simulink model "motor_sensor_PID"  (R2024b)
settings: Solver=FixedStepAuto  StartTime=0.0  StopTime=5  RelTol=1e-3  EnableMultiTasking=on
libraries: arduinolib x4, slpidlib x1, arduinosensorlib x1
settings Model: ExtModeTrigDuration=2  Creator=The MathWorks, Inc.  LastModifiedBy=davil
settings SolverCC: AlgebraicLoopSolver=TrustRegion  AutoInsertRateTranBlk=on
settings DataIOCC: ReturnWorkspaceOutputs=off
settings OptimizationCC: PassReuseOutputArgsThreshold=0  MaxStackSize=64
settings DebuggingCC: ParameterTunabilityLossMsg=error  UnconnectedInputMsg=warning  UnconnectedOutputMsg=warning  UnconnectedLineMsg=warning  ArithmeticOperatorsInVariantConditions=warning
settings HardwareCC: ProdBitPerInt=16  ProdBitPerPointer=16  ProdBitPerSizeT=16  ProdBitPerPtrDiffT=16  ProdLargestAtomicFloat=None  ProdWordSize=8  ProdHWDeviceType=Atmel->AVR  UseEmbeddedCoderFeatures=off  UseSimulinkCoderFeatures=off
settings ModelReferenceCC: EnableRefExpFcnMdlSchedulingChecks=on
settings SFSimCC: SimUseLocalCustomCode=off  MATLABDynamicMemAlloc=off  CustomCodeUndefinedFunction=UseInterfaceOnly
settings RTWCC: Description=Embedded Coder  SystemTargetFile=ert.tlc  HardwareBoard=Arduino Uno  TemplateMakefile=ert_default_tmf  GenerateReport=on  RTWUseLocalCustomCode=off  Toolchain=Arduino AVR  BuildConfiguration=Faster Runs  LaunchReport=on  GPUComputeCapability=3.5
settings CodeAppCC: ForceParamTrailComments=on  OperatorAnnotations=on
settings ERTTargetCC: ERTCustomFileBanners=off  SupportContinuousTime=on  SupportNonInlinedSFcns=on  RemoveResetFunc=off  SupportVariableSizeSignals=on  ModelStepFunctionPrototypeControlCompliant=off  ExtModeTransport=3  ExtModeStaticAlloc=on  ExtModeAutomaticAllocSize=off  ExtModeStaticAllocSize=250  ExtModeMexFile=ext_xcp  ExtModeIntrfLevel=Level2 - Open  InlinedParameterPlacement=Hierarchical  DynamicArrayContainerType=coder::array

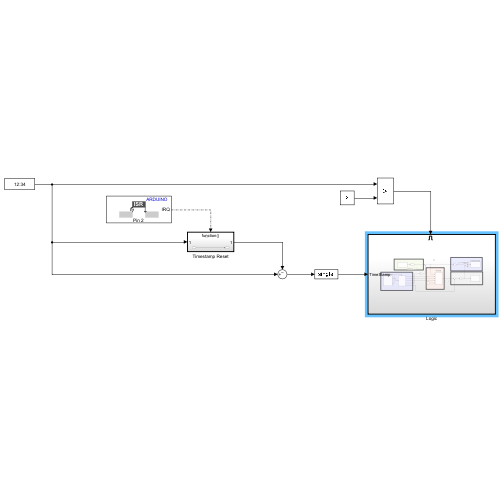
[thumbnail: Simulink's stored preview of the top-level diagram]
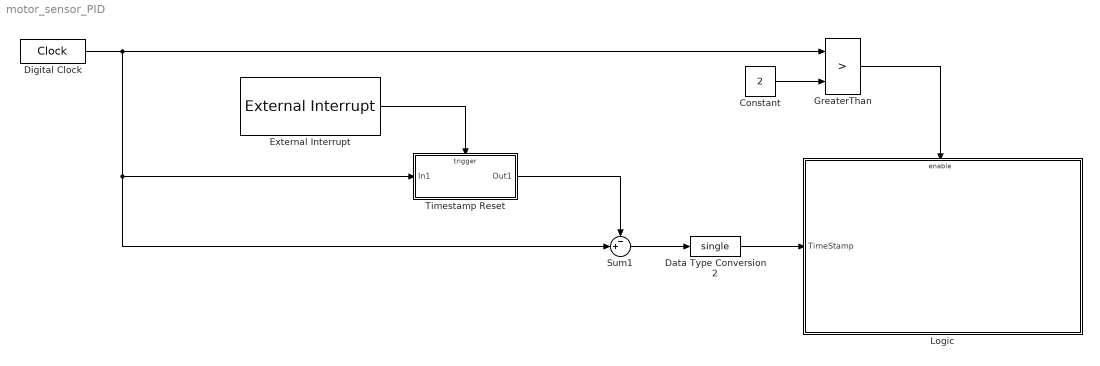
== system motor_sensor_PID ==
  Constant : Constant  Value=2
  Data Type Conversion2 : DataTypeConversion  OutDataTypeStr=single  RndMeth=Round  SaturateOnIntegerOverflow=off
  Digital Clock : DigitalClock  SampleTime=0.1
  External Interrupt : arduinolib/External Interrupt  Pin=2  PullUp=off  Mode=RISING  InterruptSimulationInput=off
  GreaterThan : RelationalOperator  Operator=>  OutDataTypeStr=boolean  RndMeth=Simplest  InputSameDT=off
  Logic : Subsystem
  Sum1 : Sum  Inputs=-+|
  Timestamp Reset : Subsystem  TreatAsAtomicUnit=on
  wires:
  GreaterThan/1 -> Logic/Enable
  Constant/1 -> GreaterThan/2
  Digital Clock/1 -> GreaterThan/1, Timestamp Reset/1(In1), Sum1/2
  Sum1/1 -> Data Type Conversion2/1
  Timestamp Reset/1(Out1) -> Sum1/1
  External Interrupt/1 -> Timestamp Reset/Trigger
  Data Type Conversion2/1 -> Logic/1(TimeStamp)

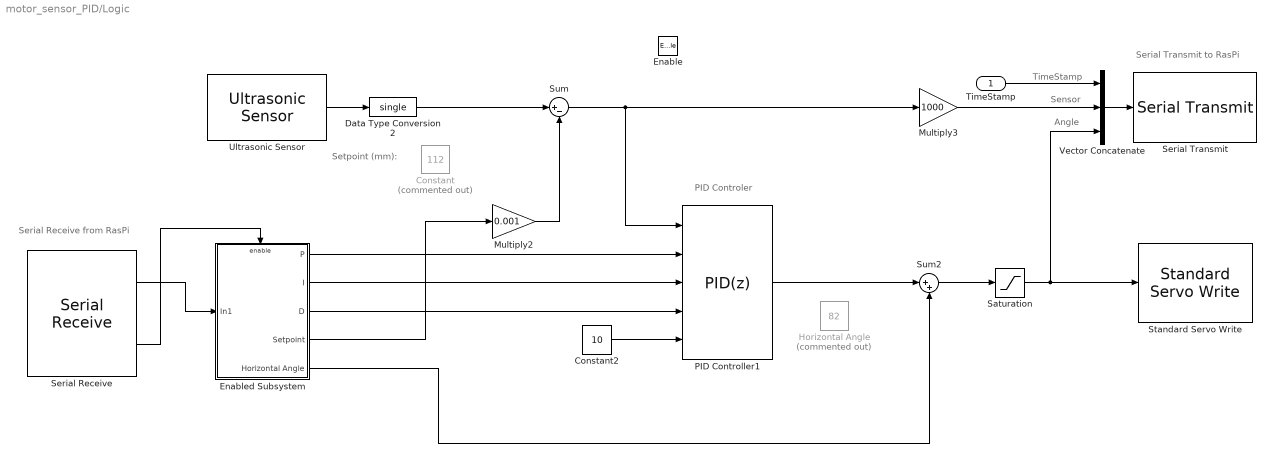
== system motor_sensor_PID/Logic ==
  note: Setpoint (mm):
  note: Serial Receive from RasPi
  note: PID Controler
  note: Serial Transmit to RasPi
  note: TimeStamp
  note: Sensor
  note: Angle
  TimeStamp : Inport
  Enable : EnablePort
  Constant : Constant  Commented=on  Value=112  OutDataTypeStr=single
  Constant2 : Constant  Value=10  OutDataTypeStr=single
  Data Type Conversion2 : DataTypeConversion  OutDataTypeStr=single  RndMeth=Round  SaturateOnIntegerOverflow=off
  Enabled Subsystem : Subsystem  TreatAsAtomicUnit=on
  Horizontal Angle : Constant  Commented=on  Value=82  OutDataTypeStr=single
  Multiply2 : Gain  Gain=0.001
  Multiply3 : Gain  Gain=1000
  PID Controller1 : slpidlib/PID Controller  Controller=PID  Form=Parallel  TimeDomain=Discrete-time  UseExternalTs=off  SampleTime=-1  IntegratorMethod=Forward Euler  FilterMethod=Forward Euler  ControllerParametersSource=external  P=1  I=1  UseKiTs=off  D=0  UseExternalDerivativeSource=off  N=100  UseFilter=on  TunerSelectOption=Transfer Function Based (PID Tuner App)  InitialConditionSource=internal  InitialConditionForIntegrator=0  InitialConditionForFilter=0  DifferentiatorICPrevScaledInput=0  ExternalReset=none  TrackingMode=off  Kt=1  LimitOutput=off  SatLimitsSource=internal  UpperSaturationLimit=180  LowerSaturationLimit=0  LinearizeAsGain=on  AntiWindupMode=none  Kb=1  LimitIntegrator=off  UpperIntegratorSaturationLimit=inf  LowerIntegratorSaturationLimit=-inf  POutMin=[]  POutMax=[]  IOutMin=[]  IOutMax=[]  DOutMin=[]  DOutMax=[]  NOutMin=[]  NOutMax=[]  SumOutMin=[]  SumOutMax=[]  SaturationOutMin=[]  SaturationOutMax=[]  PParamMin=[]  PParamMax=[]  IParamMin=[]  IParamMax=[]  DParamMin=[]  DParamMax=[]  NParamMin=[]  NParamMax=[]  KbParamMin=[]  KbParamMax=[]  KtParamMin=[]  KtParamMax=[]  KbOutMin=[]  KbOutMax=[]  KtOutMin=[]  KtOutMax=[]  IntegratorOutMin=[]  IntegratorOutMax=[]  FilterOutMin=[]  FilterOutMax=[]  SumI1OutMin=[]  SumI1OutMax=[]  SumI2OutMin=[]  SumI2OutMax=[]  SumI3OutMin=[]  SumI3OutMax=[]  SumI4OutMin=[]  SumI4OutMax=[]  SumDOutMin=[]  SumDOutMax=[]  DifferentiatorOutMin=[]  DifferentiatorOutMax=[]  FilterDiffOutCoefMin=[]  FilterDiffOutCoefMax=[]  ReciprocalOutMin=[]  ReciprocalOutMax=[]  SumDenOutMin=[]  SumDenOutMax=[]  SumNumOutMin=[]  SumNumOutMax=[]  DivideOutMin=[]  DivideOutMax=[]  UdiffTsProdOutMin=[]  UdiffTsProdOutMax=[]  NTsProdOutMin=[]  NTsProdOutMax=[]  UintegralTsProdOutMin=[]  UintegralTsProdOutMax=[]  UngainTsProdOutMin=[]  UngainTsProdOutMax=[]  ClampingZeroOutDataTypeStr=Inherit: Inherit via back propagation  ClampingZeroOutMin=[]  ClampingZeroOutMax=[]  FilterDenConstantOutDataTypeStr=Inherit: Inherit via back propagation  FilterDenConstantOutMin=[]  FilterDenConstantOutMax=[]  PCopyOutDataTypeStr=Inherit: Inherit via back propagation  PCopyOutMin=[]  PCopyOutMax=[]  NCopyOutDataTypeStr=Inherit: Inherit via back propagation  NCopyOutMin=[]  NCopyOutMax=[]  IntegratorContinuousStateAttributes=''  IntegratorStateMustResolveToSignalObject=off  IntegratorRTWStateStorageClass=Auto  FilterContinuousStateAttributes=''  FilterStateMustResolveToSignalObject=off  FilterRTWStateStorageClass=Auto  ParallelPVariant=ExternalParameters  IdealPVariant=Disabled  IVariant=ExternalParameters  DVariant=ExternalParameters  IntegratorVariant=Discrete  SatVariant=Disabled  AWVariant=Passthrough  PCopyVariant=Disabled  TRVariant=Disabled  FdbkBlocksVariant=Forward  IdealPFdbkVariant=Disabled  SatFdbkVariant=Disabled  DerivativeFilterVariant=ForwardEulerFilter  NVariant=ExternalParameters  NCopyVariant=Disabled  FilterICVariant=InternalICsFilter  IntegratorICVariant=InternalICs  ExternalResetVariant=Disabled  TRSumVariant=Passthrough  SumFdbkVariant=Disabled  SumVariant=Sum_PID  TsampFilterVariant=InternalTs  TsampNgainVariant=Passthrough  TsampIntegralVariant=Disabled_SignalSpec  ExternalSaturationOutDataTypeStr=Inherit: Same as second input  DerivativeSourceVariant=ErrorSignal  PreIntVariant=InternalPreInt
  Saturation : Saturate  UpperLimit=180  LowerLimit=0
  Serial Receive : arduinolib/Serial Receive  portNumber=0  DataType=single  blockPlatform=ARDUINO  TimeOut=0  MaxDataLength=10  isARMArch=off  DataLengthOption=Length via dialog  Datalength=5  Header=[]  Terminator=[]  SampleTime=0.1  ShowOutStatus=on
  Serial Transmit : arduinolib/Serial Transmit  portNumber=0  sendmode=write  sendformat=Decimal  floatprecision=4  header=[]  terminator=[]  blockPlatform=ARDUINO
  Standard Servo Write : arduinolib/Standard Servo Write  pinNumber=4  ServoIndex=0  blockPlatform=ARDUINO
  Sum : Sum  Inputs=|+-
  Sum2 : Sum  Inputs=|++
  Ultrasonic Sensor : arduinosensorlib/Ultrasonic Sensor  NumSignalPins=2  TrigPin=7  EchoPin=6  SignalPin=3  SampleTime_=0.1  blockPlatform=ARDUINO
  Vector Concatenate : Concatenate  NumInputs=3
  wires:
  Enabled Subsystem/4(Setpoint) -> Multiply2/1
  Serial Receive/1 -> Enabled Subsystem/1(In1)
  Enabled Subsystem/5(Horizontal Angle) -> Sum2/2
  Serial Receive/2 -> Enabled Subsystem/Enable
  Data Type Conversion2/1 -> Sum/1
  Saturation/1 -> Standard Servo Write/1, Vector Concatenate/3
  Multiply3/1 -> Vector Concatenate/2
  Sum2/1 -> Saturation/1
  PID Controller1/1 -> Sum2/1
  Sum/1 -> PID Controller1/1, Multiply3/1
  Ultrasonic Sensor/1 -> Data Type Conversion2/1
  Constant2/1 -> PID Controller1/5
  Multiply2/1 -> Sum/2
  Vector Concatenate/1 -> Serial Transmit/1
  TimeStamp/1 -> Vector Concatenate/1
  Enabled Subsystem/1(P) -> PID Controller1/2
  Enabled Subsystem/2(I) -> PID Controller1/3
  Enabled Subsystem/3(D) -> PID Controller1/4

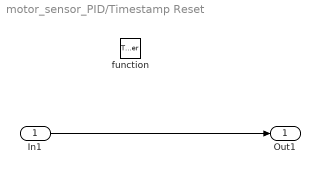
== system motor_sensor_PID/Timestamp Reset ==
  In1 : Inport
  function : TriggerPort  TriggerType=function-call  VariantControl=(inherit)
  Out1 : Outport
  wires:
  In1/1 -> Out1/1

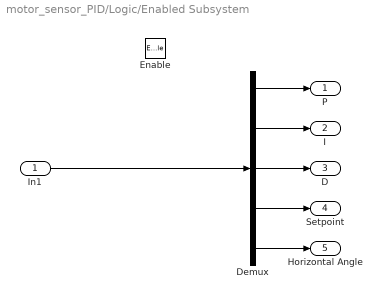
== system motor_sensor_PID/Logic/Enabled Subsystem ==
  In1 : Inport
  Enable : EnablePort
  Demux : Demux  Outputs=5
  P : Outport
  I : Outport  Port=2
  D : Outport  Port=3
  Setpoint : Outport  Port=4
  Horizontal Angle : Outport  Port=5
  wires:
  In1/1 -> Demux/1
  Demux/1 -> P/1
  Demux/2 -> I/1
  Demux/3 -> D/1
  Demux/4 -> Setpoint/1
  Demux/5 -> Horizontal Angle/1
